simulink model "ALU"  (R2021a)
settings: Solver=VariableStepAuto  StartTime=0.0  StopTime=10.0  RelTol=1e-3
settings Model: Creator=kbhar  LastModifiedBy=kbhar

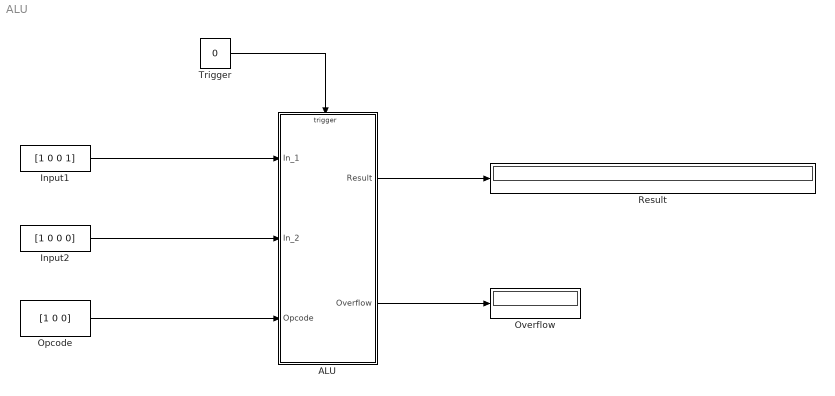
== system ALU ==
  ALU : Subsystem
  Input1 : Constant  Value=[1 0 0 1]
  Input2 : Constant  Value=[1 0 0 0]
  Opcode : Constant  Value=[1 0 0]
  Overflow : Display
  Result : Display
  Trigger : Constant  Value=0
  wires:
  Input2/1 -> ALU/2(In_2)
  Input1/1 -> ALU/1(In_1)
  Opcode/1 -> ALU/3(Opcode)
  ALU/1(Result) -> Result/1
  ALU/2(Overflow) -> Overflow/1
  Trigger/1 -> ALU/Trigger

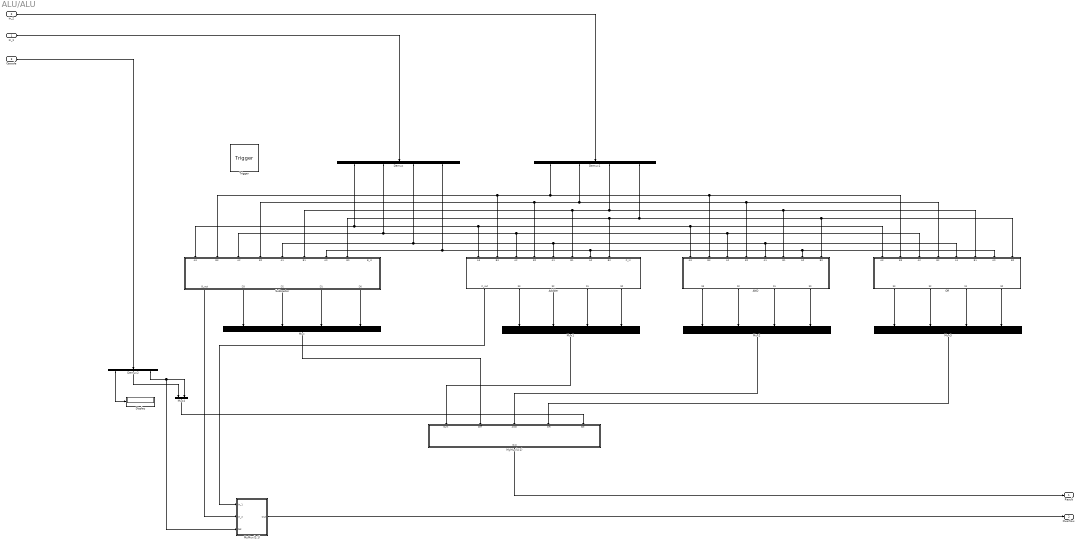
== system ALU/ALU ==
  In_1 : Inport
  In_2 : Inport  Port=2
  Opcode : Inport  Port=3
  Trigger : TriggerPort  VariantControl=(inherit)  PortDimensions=1
  AND : Subsystem
  Addder : Subsystem
  Demux : Demux
  Demux1 : Demux
  Demux2 : Demux  Outputs=3
  Display : Display
  Mux{,1..3} (4 alike) : Mux
  Mux4 : Mux  Inputs=2
  MyMux(2:1) : Subsystem
  MyMux(4:1) : Subsystem
  OR : Subsystem
  Subtractor : Subsystem
  Result : Outport
  Overflow : Outport  Port=2
  wires:
  AND/2(S2) -> Mux2/2
  Demux1/3 -> OR/6(B1), AND/6(B1), Subtractor/6(B1), Addder/6(B1)
  OR/1(S3) -> Mux3/1
  Subtractor/5(D0) -> Mux/4
  OR/3(S1) -> Mux3/3
  Demux1/2 -> OR/4(B2), AND/4(B2), Subtractor/4(B2), Addder/4(B2)
  Mux/1 -> MyMux(4:1)/2(Diff)
  Demux/4 -> Subtractor/7(A0), OR/7(A0), AND/7(A0), Addder/7(A0)
  Addder/3(S2) -> Mux1/2
  Subtractor/2(D3) -> Mux/1
  Demux1/4 -> Subtractor/8(B0), Addder/8(B0), OR/8(B0), AND/8(B0)
  Demux/2 -> Subtractor/3(A2), OR/3(A2), AND/3(A2), Addder/3(A2)
  Demux/1 -> Subtractor/1(A3), OR/1(A3), AND/1(A3), Addder/1(A3)
  MyMux(2:1)/1(Out) -> Overflow/1
  Subtractor/1(B_out) -> MyMux(2:1)/2(In_2)
  Demux1/1 -> OR/2(B3), AND/2(B3), Subtractor/2(B3), Addder/2(B3)
  Demux/3 -> Subtractor/5(A1), AND/5(A1), OR/5(A1), Addder/5(A1)
  MyMux(4:1)/1(Out) -> Result/1
  Subtractor/3(D2) -> Mux/2
  Mux3/1 -> MyMux(4:1)/4(OR)
  Subtractor/4(D1) -> Mux/3
  Mux1/1 -> MyMux(4:1)/1(Sum)
  ? -> Addder/9(C_in)
  AND/1(S3) -> Mux2/1
  Mux2/1 -> MyMux(4:1)/3(AND)
  In_2/1 -> Demux1/1
  OR/2(S2) -> Mux3/2
  Mux4/1 -> MyMux(4:1)/5(Sel)
  AND/4(S0) -> Mux2/4
  Demux2/1 -> Display/1
  Demux2/3 -> MyMux(2:1)/3(Sel), Mux4/2
  Demux2/2 -> Mux4/1
  Addder/1(C_out) -> MyMux(2:1)/1(In_1)
  Addder/4(S1) -> Mux1/3
  AND/3(S1) -> Mux2/3
  Addder/5(S0) -> Mux1/4
  OR/4(S0) -> Mux3/4
  ? -> Subtractor/9(B_in)
  Addder/2(S3) -> Mux1/1
  Opcode/1 -> Demux2/1
  In_1/1 -> Demux/1

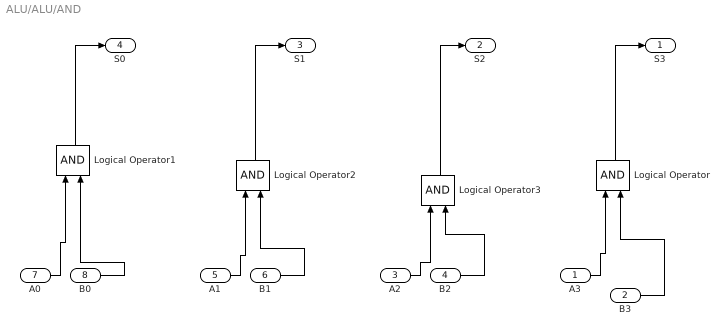
== system ALU/ALU/AND ==
  A3 : Inport
  B3 : Inport  Port=2
  A2 : Inport  Port=3
  B2 : Inport  Port=4
  A1 : Inport  Port=5
  B1 : Inport  Port=6
  A0 : Inport  Port=7
  B0 : Inport  Port=8
  Logical Operator{,1..3} (4 alike) : Logic  AllPortsSameDT=off  OutDataTypeStr=boolean
  S3 : Outport
  S2 : Outport  Port=2
  S1 : Outport  Port=3
  S0 : Outport  Port=4
  wires:
  Logical Operator2/1 -> S1/1
  B1/1 -> Logical Operator2/2
  A1/1 -> Logical Operator2/1
  A2/1 -> Logical Operator3/1
  B0/1 -> Logical Operator1/2
  B3/1 -> Logical Operator/2
  B2/1 -> Logical Operator3/2
  A0/1 -> Logical Operator1/1
  A3/1 -> Logical Operator/1
  Logical Operator3/1 -> S2/1
  Logical Operator1/1 -> S0/1
  Logical Operator/1 -> S3/1

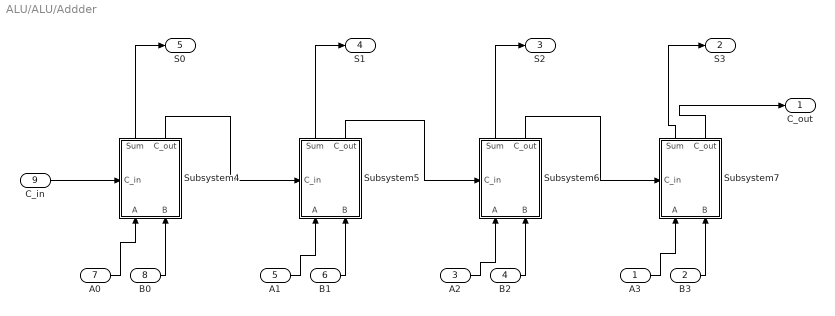
== system ALU/ALU/Addder ==
  A3 : Inport
  B3 : Inport  Port=2
  A2 : Inport  Port=3
  B2 : Inport  Port=4
  A1 : Inport  Port=5
  B1 : Inport  Port=6
  A0 : Inport  Port=7
  B0 : Inport  Port=8
  C_in : Inport  Port=9
  Subsystem4 : Subsystem
      settings: PortSchema="{\"entries\":[{\"content\":{\"sides\":[{\"content\":{\"connectorIds\":[\"In1\",\"In2\"]},\"type\":\"ConnectorPlacement.EquallySpacedRectSide\",\"uuid\":\"38d1d783-1e84-469f-b88f-34400794f458\"},{\"content\":{\"connectorIds\":[\"Out1\",\"Out2\"],\"side\":\"RIGHT\"},\"type\":\"ConnectorPlacement.EquallySpacedRectSide\",\"uuid\":\"9549b396-3b16-432f-9c12-dae7a5b8dc11\"},{\"content\":{\"connectorIds\":[\"In3\"],\"side\":\"TOP\"},\"type\":\"ConnectorPlacement.EquallySpacedRectSide\",\"uuid\":\"526a5790-86b3-4626-b4aa-b9520108ec40\"}]},\"type\":\"ConnectorPlacement.EquallySpacedConnector\",\"uuid\":\"b57ea0ad-738f-4734-9daa-a65058de1f48\"}],\"packageUris\":[\"http://schema.mathworks.com/mf0/Connector/R2020b\"],\"version\":\"1.0\"}"
  Subsystem5 : Subsystem
      settings: PortSchema="{\"entries\":[{\"content\":{\"sides\":[{\"content\":{\"connectorIds\":[\"In1\",\"In2\"]},\"type\":\"ConnectorPlacement.EquallySpacedRectSide\",\"uuid\":\"38d1d783-1e84-469f-b88f-34400794f458\"},{\"content\":{\"connectorIds\":[\"Out1\",\"Out2\"],\"side\":\"RIGHT\"},\"type\":\"ConnectorPlacement.EquallySpacedRectSide\",\"uuid\":\"9549b396-3b16-432f-9c12-dae7a5b8dc11\"},{\"content\":{\"connectorIds\":[\"In3\"],\"side\":\"TOP\"},\"type\":\"ConnectorPlacement.EquallySpacedRectSide\",\"uuid\":\"526a5790-86b3-4626-b4aa-b9520108ec40\"}]},\"type\":\"ConnectorPlacement.EquallySpacedConnector\",\"uuid\":\"b57ea0ad-738f-4734-9daa-a65058de1f48\"}],\"packageUris\":[\"http://schema.mathworks.com/mf0/Connector/R2020b\"],\"version\":\"1.0\"}"
  Subsystem6 : Subsystem
      settings: PortSchema="{\"entries\":[{\"content\":{\"sides\":[{\"content\":{\"connectorIds\":[\"In1\",\"In2\"]},\"type\":\"ConnectorPlacement.EquallySpacedRectSide\",\"uuid\":\"38d1d783-1e84-469f-b88f-34400794f458\"},{\"content\":{\"connectorIds\":[\"Out1\",\"Out2\"],\"side\":\"RIGHT\"},\"type\":\"ConnectorPlacement.EquallySpacedRectSide\",\"uuid\":\"9549b396-3b16-432f-9c12-dae7a5b8dc11\"},{\"content\":{\"connectorIds\":[\"In3\"],\"side\":\"TOP\"},\"type\":\"ConnectorPlacement.EquallySpacedRectSide\",\"uuid\":\"526a5790-86b3-4626-b4aa-b9520108ec40\"}]},\"type\":\"ConnectorPlacement.EquallySpacedConnector\",\"uuid\":\"b57ea0ad-738f-4734-9daa-a65058de1f48\"}],\"packageUris\":[\"http://schema.mathworks.com/mf0/Connector/R2020b\"],\"version\":\"1.0\"}"
  Subsystem7 : Subsystem
      settings: PortSchema="{\"entries\":[{\"content\":{\"sides\":[{\"content\":{\"connectorIds\":[\"In1\",\"In2\"]},\"type\":\"ConnectorPlacement.EquallySpacedRectSide\",\"uuid\":\"38d1d783-1e84-469f-b88f-34400794f458\"},{\"content\":{\"connectorIds\":[\"Out1\",\"Out2\"],\"side\":\"RIGHT\"},\"type\":\"ConnectorPlacement.EquallySpacedRectSide\",\"uuid\":\"9549b396-3b16-432f-9c12-dae7a5b8dc11\"},{\"content\":{\"connectorIds\":[\"In3\"],\"side\":\"TOP\"},\"type\":\"ConnectorPlacement.EquallySpacedRectSide\",\"uuid\":\"526a5790-86b3-4626-b4aa-b9520108ec40\"}]},\"type\":\"ConnectorPlacement.EquallySpacedConnector\",\"uuid\":\"b57ea0ad-738f-4734-9daa-a65058de1f48\"}],\"packageUris\":[\"http://schema.mathworks.com/mf0/Connector/R2020b\"],\"version\":\"1.0\"}"
  C_out : Outport
  S3 : Outport  Port=2
  S2 : Outport  Port=3
  S1 : Outport  Port=4
  S0 : Outport  Port=5
  wires:
  Subsystem5/2(C_out) -> Subsystem6/3(C_in)
  Subsystem5/1(Sum) -> S1/1
  Subsystem7/2(C_out) -> C_out/1
  B1/1 -> Subsystem5/2(B)
  Subsystem6/2(C_out) -> Subsystem7/3(C_in)
  A1/1 -> Subsystem5/1(A)
  A2/1 -> Subsystem6/1(A)
  Subsystem4/2(C_out) -> Subsystem5/3(C_in)
  B0/1 -> Subsystem4/2(B)
  B3/1 -> Subsystem7/2(B)
  B2/1 -> Subsystem6/2(B)
  A0/1 -> Subsystem4/1(A)
  A3/1 -> Subsystem7/1(A)
  Subsystem6/1(Sum) -> S2/1
  C_in/1 -> Subsystem4/3(C_in)
  Subsystem4/1(Sum) -> S0/1
  Subsystem7/1(Sum) -> S3/1

== system ALU/ALU/MyMux(2:1) ==
  In_1 : Inport
  In_2 : Inport  Port=2
  Sel : Inport  Port=3
  Logical Operator : Logic  AllPortsSameDT=off  OutDataTypeStr=boolean
  Logical Operator1 : Logic  Operator=NOT  AllPortsSameDT=off  OutDataTypeStr=boolean
  Logical Operator2 : Logic  AllPortsSameDT=off  OutDataTypeStr=boolean
  Logical Operator3 : Logic  Operator=OR  AllPortsSameDT=off  OutDataTypeStr=boolean
  Out : Outport
  wires:
  Logical Operator1/1 -> Logical Operator/2
  In_1/1 -> Logical Operator/1
  Logical Operator2/1 -> Logical Operator3/2
  Sel/1 -> Logical Operator1/1, Logical Operator2/2
  Logical Operator3/1 -> Out/1
  In_2/1 -> Logical Operator2/1
  Logical Operator/1 -> Logical Operator3/1

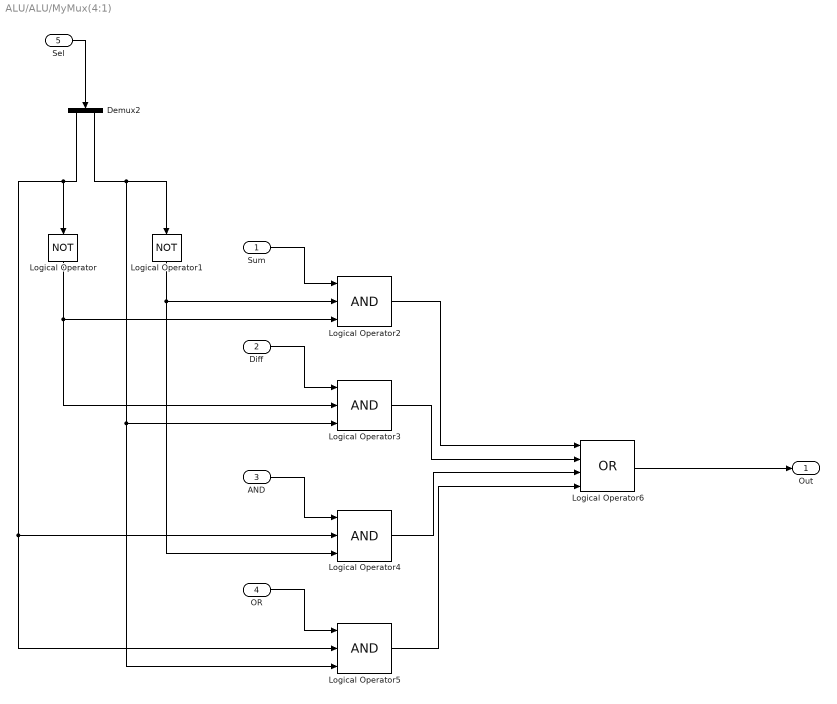
== system ALU/ALU/MyMux(4:1) ==
  Sum : Inport
  Diff : Inport  Port=2
  AND : Inport  Port=3
  OR : Inport  Port=4
  Sel : Inport  Port=5
  Demux2 : Demux  Outputs=2
  Logical Operator : Logic  Operator=NOT  AllPortsSameDT=off  OutDataTypeStr=boolean
  Logical Operator1 : Logic  Operator=NOT  AllPortsSameDT=off  OutDataTypeStr=boolean
  Logical Operator{2..5} (4 alike) : Logic  Inputs=3  AllPortsSameDT=off  OutDataTypeStr=boolean
  Logical Operator6 : Logic  Operator=OR  Inputs=4  AllPortsSameDT=off  OutDataTypeStr=boolean
  Out : Outport
  wires:
  Demux2/1 -> Logical Operator4/2, Logical Operator5/2, Logical Operator/1
  Demux2/2 -> Logical Operator5/3, Logical Operator3/3, Logical Operator1/1
  Logical Operator1/1 -> Logical Operator2/2, Logical Operator4/3
  Logical Operator2/1 -> Logical Operator6/1
  Logical Operator3/1 -> Logical Operator6/2
  Logical Operator/1 -> Logical Operator2/3, Logical Operator3/2
  Logical Operator4/1 -> Logical Operator6/3
  Logical Operator5/1 -> Logical Operator6/4
  Diff/1 -> Logical Operator3/1
  AND/1 -> Logical Operator4/1
  OR/1 -> Logical Operator5/1
  Sum/1 -> Logical Operator2/1
  Logical Operator6/1 -> Out/1
  Sel/1 -> Demux2/1

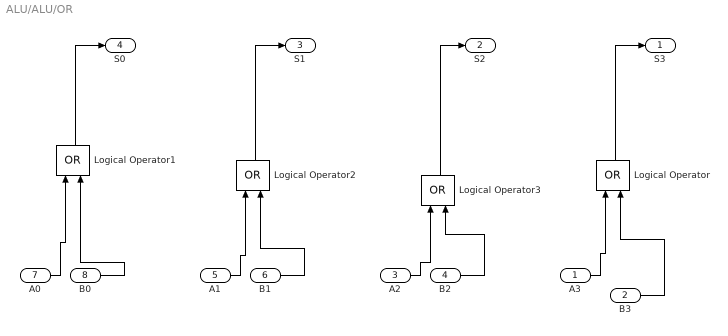
== system ALU/ALU/OR ==
  A3 : Inport
  B3 : Inport  Port=2
  A2 : Inport  Port=3
  B2 : Inport  Port=4
  A1 : Inport  Port=5
  B1 : Inport  Port=6
  A0 : Inport  Port=7
  B0 : Inport  Port=8
  Logical Operator{,1..3} (4 alike) : Logic  Operator=OR  AllPortsSameDT=off  OutDataTypeStr=boolean
  S3 : Outport
  S2 : Outport  Port=2
  S1 : Outport  Port=3
  S0 : Outport  Port=4
  wires:
  Logical Operator2/1 -> S1/1
  B1/1 -> Logical Operator2/2
  A1/1 -> Logical Operator2/1
  A2/1 -> Logical Operator3/1
  B0/1 -> Logical Operator1/2
  B3/1 -> Logical Operator/2
  B2/1 -> Logical Operator3/2
  A0/1 -> Logical Operator1/1
  A3/1 -> Logical Operator/1
  Logical Operator3/1 -> S2/1
  Logical Operator1/1 -> S0/1
  Logical Operator/1 -> S3/1

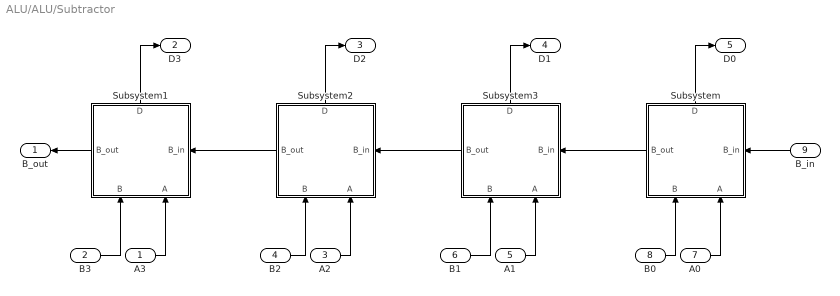
== system ALU/ALU/Subtractor ==
  A3 : Inport
  B3 : Inport  Port=2
  A2 : Inport  Port=3
  B2 : Inport  Port=4
  A1 : Inport  Port=5
  B1 : Inport  Port=6
  A0 : Inport  Port=7
  B0 : Inport  Port=8
  B_in : Inport  Port=9
  Subsystem : Subsystem
      settings: PortSchema="{\"entries\":[{\"content\":{\"sides\":[{\"content\":{\"connectorIds\":[\"In1\",\"In2\"]},\"type\":\"ConnectorPlacement.EquallySpacedRectSide\",\"uuid\":\"38d1d783-1e84-469f-b88f-34400794f458\"},{\"content\":{\"connectorIds\":[\"Out1\"],\"side\":\"RIGHT\"},\"type\":\"ConnectorPlacement.EquallySpacedRectSide\",\"uuid\":\"9549b396-3b16-432f-9c12-dae7a5b8dc11\"},{\"content\":{\"connectorIds\":[\"Out2\"],\"side\":\"TOP\"},\"type\":\"ConnectorPlacement.EquallySpacedRectSide\",\"uuid\":\"526a5790-86b3-4626-b4aa-b9520108ec40\"},{\"content\":{\"connectorIds\":[\"In3\"],\"side\":\"BOTTOM\"},\"type\":\"ConnectorPlacement.EquallySpacedRectSide\",\"uuid\":\"7b9a1b6a-14be-425f-b6da-6563ee756159\"}]},\"type\":\"ConnectorPlacement.EquallySpacedConnector\",\"uuid\":\"b57ea0ad-738f-4734-9daa-a65058de1f48\"}],\"packageUris\":[\"http://schema.mathworks.com/mf0/Connector/R2020b\"],\"version\":\"1.0\"}"
  Subsystem1 : Subsystem
      settings: PortSchema="{\"entries\":[{\"content\":{\"sides\":[{\"content\":{\"connectorIds\":[\"In1\",\"In2\"]},\"type\":\"ConnectorPlacement.EquallySpacedRectSide\",\"uuid\":\"38d1d783-1e84-469f-b88f-34400794f458\"},{\"content\":{\"connectorIds\":[\"Out1\"],\"side\":\"RIGHT\"},\"type\":\"ConnectorPlacement.EquallySpacedRectSide\",\"uuid\":\"9549b396-3b16-432f-9c12-dae7a5b8dc11\"},{\"content\":{\"connectorIds\":[\"Out2\"],\"side\":\"TOP\"},\"type\":\"ConnectorPlacement.EquallySpacedRectSide\",\"uuid\":\"526a5790-86b3-4626-b4aa-b9520108ec40\"},{\"content\":{\"connectorIds\":[\"In3\"],\"side\":\"BOTTOM\"},\"type\":\"ConnectorPlacement.EquallySpacedRectSide\",\"uuid\":\"7b9a1b6a-14be-425f-b6da-6563ee756159\"}]},\"type\":\"ConnectorPlacement.EquallySpacedConnector\",\"uuid\":\"b57ea0ad-738f-4734-9daa-a65058de1f48\"}],\"packageUris\":[\"http://schema.mathworks.com/mf0/Connector/R2020b\"],\"version\":\"1.0\"}"
  Subsystem2 : Subsystem
      settings: PortSchema="{\"entries\":[{\"content\":{\"sides\":[{\"content\":{\"connectorIds\":[\"In1\",\"In2\"]},\"type\":\"ConnectorPlacement.EquallySpacedRectSide\",\"uuid\":\"38d1d783-1e84-469f-b88f-34400794f458\"},{\"content\":{\"connectorIds\":[\"Out1\"],\"side\":\"RIGHT\"},\"type\":\"ConnectorPlacement.EquallySpacedRectSide\",\"uuid\":\"9549b396-3b16-432f-9c12-dae7a5b8dc11\"},{\"content\":{\"connectorIds\":[\"Out2\"],\"side\":\"TOP\"},\"type\":\"ConnectorPlacement.EquallySpacedRectSide\",\"uuid\":\"526a5790-86b3-4626-b4aa-b9520108ec40\"},{\"content\":{\"connectorIds\":[\"In3\"],\"side\":\"BOTTOM\"},\"type\":\"ConnectorPlacement.EquallySpacedRectSide\",\"uuid\":\"7b9a1b6a-14be-425f-b6da-6563ee756159\"}]},\"type\":\"ConnectorPlacement.EquallySpacedConnector\",\"uuid\":\"b57ea0ad-738f-4734-9daa-a65058de1f48\"}],\"packageUris\":[\"http://schema.mathworks.com/mf0/Connector/R2020b\"],\"version\":\"1.0\"}"
  Subsystem3 : Subsystem
      settings: PortSchema="{\"entries\":[{\"content\":{\"sides\":[{\"content\":{\"connectorIds\":[\"In1\",\"In2\"]},\"type\":\"ConnectorPlacement.EquallySpacedRectSide\",\"uuid\":\"38d1d783-1e84-469f-b88f-34400794f458\"},{\"content\":{\"connectorIds\":[\"Out1\"],\"side\":\"RIGHT\"},\"type\":\"ConnectorPlacement.EquallySpacedRectSide\",\"uuid\":\"9549b396-3b16-432f-9c12-dae7a5b8dc11\"},{\"content\":{\"connectorIds\":[\"Out2\"],\"side\":\"TOP\"},\"type\":\"ConnectorPlacement.EquallySpacedRectSide\",\"uuid\":\"526a5790-86b3-4626-b4aa-b9520108ec40\"},{\"content\":{\"connectorIds\":[\"In3\"],\"side\":\"BOTTOM\"},\"type\":\"ConnectorPlacement.EquallySpacedRectSide\",\"uuid\":\"7b9a1b6a-14be-425f-b6da-6563ee756159\"}]},\"type\":\"ConnectorPlacement.EquallySpacedConnector\",\"uuid\":\"b57ea0ad-738f-4734-9daa-a65058de1f48\"}],\"packageUris\":[\"http://schema.mathworks.com/mf0/Connector/R2020b\"],\"version\":\"1.0\"}"
  B_out : Outport
  D3 : Outport  Port=2
  D2 : Outport  Port=3
  D1 : Outport  Port=4
  D0 : Outport  Port=5
  wires:
  B_in/1 -> Subsystem/3(B_in)
  Subsystem3/2(B_out) -> Subsystem2/3(B_in)
  Subsystem2/2(B_out) -> Subsystem1/3(B_in)
  Subsystem/2(B_out) -> Subsystem3/3(B_in)
  Subsystem1/2(B_out) -> B_out/1
  A0/1 -> Subsystem/2(A)
  B0/1 -> Subsystem/1(B)
  B3/1 -> Subsystem1/1(B)
  A3/1 -> Subsystem1/2(A)
  A1/1 -> Subsystem3/2(A)
  B1/1 -> Subsystem3/1(B)
  B2/1 -> Subsystem2/1(B)
  A2/1 -> Subsystem2/2(A)
  Subsystem1/1(D) -> D3/1
  Subsystem/1(D) -> D0/1
  Subsystem3/1(D) -> D1/1
  Subsystem2/1(D) -> D2/1

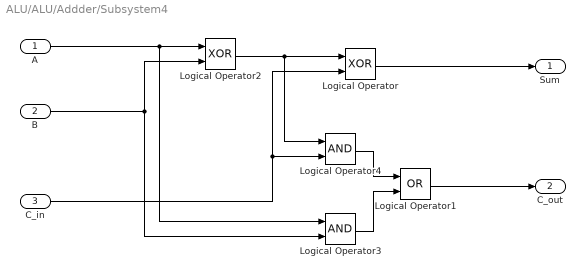
== system ALU/ALU/Addder/Subsystem4 ==
  A : Inport
  B : Inport  Port=2
  C_in : Inport  Port=3
  Logical Operator : Logic  Operator=XOR  AllPortsSameDT=off  OutDataTypeStr=boolean
  Logical Operator1 : Logic  Operator=OR  AllPortsSameDT=off  OutDataTypeStr=boolean
  Logical Operator2 : Logic  Operator=XOR  AllPortsSameDT=off  OutDataTypeStr=boolean
  Logical Operator3 : Logic  AllPortsSameDT=off  OutDataTypeStr=boolean
  Logical Operator4 : Logic  AllPortsSameDT=off  OutDataTypeStr=boolean
  Sum : Outport
  C_out : Outport  Port=2
  wires:
  B/1 -> Logical Operator3/2, Logical Operator2/2
  A/1 -> Logical Operator3/1, Logical Operator2/1
  Logical Operator4/1 -> Logical Operator1/1
  Logical Operator/1 -> Sum/1
  Logical Operator2/1 -> Logical Operator4/1, Logical Operator/1
  C_in/1 -> Logical Operator4/2, Logical Operator/2
  Logical Operator3/1 -> Logical Operator1/2
  Logical Operator1/1 -> C_out/1

== system ALU/ALU/Addder/Subsystem5 ==
  A : Inport
  B : Inport  Port=2
  C_in : Inport  Port=3
  Logical Operator : Logic  Operator=XOR  AllPortsSameDT=off  OutDataTypeStr=boolean
  Logical Operator1 : Logic  Operator=OR  AllPortsSameDT=off  OutDataTypeStr=boolean
  Logical Operator2 : Logic  Operator=XOR  AllPortsSameDT=off  OutDataTypeStr=boolean
  Logical Operator3 : Logic  AllPortsSameDT=off  OutDataTypeStr=boolean
  Logical Operator4 : Logic  AllPortsSameDT=off  OutDataTypeStr=boolean
  Sum : Outport
  C_out : Outport  Port=2
  wires:
  B/1 -> Logical Operator3/2, Logical Operator2/2
  A/1 -> Logical Operator3/1, Logical Operator2/1
  Logical Operator4/1 -> Logical Operator1/1
  Logical Operator/1 -> Sum/1
  Logical Operator2/1 -> Logical Operator4/1, Logical Operator/1
  C_in/1 -> Logical Operator4/2, Logical Operator/2
  Logical Operator3/1 -> Logical Operator1/2
  Logical Operator1/1 -> C_out/1

== system ALU/ALU/Addder/Subsystem6 ==
  A : Inport
  B : Inport  Port=2
  C_in : Inport  Port=3
  Logical Operator : Logic  Operator=XOR  AllPortsSameDT=off  OutDataTypeStr=boolean
  Logical Operator1 : Logic  Operator=OR  AllPortsSameDT=off  OutDataTypeStr=boolean
  Logical Operator2 : Logic  Operator=XOR  AllPortsSameDT=off  OutDataTypeStr=boolean
  Logical Operator3 : Logic  AllPortsSameDT=off  OutDataTypeStr=boolean
  Logical Operator4 : Logic  AllPortsSameDT=off  OutDataTypeStr=boolean
  Sum : Outport
  C_out : Outport  Port=2
  wires:
  B/1 -> Logical Operator3/2, Logical Operator2/2
  A/1 -> Logical Operator3/1, Logical Operator2/1
  Logical Operator4/1 -> Logical Operator1/1
  Logical Operator/1 -> Sum/1
  Logical Operator2/1 -> Logical Operator4/1, Logical Operator/1
  C_in/1 -> Logical Operator4/2, Logical Operator/2
  Logical Operator3/1 -> Logical Operator1/2
  Logical Operator1/1 -> C_out/1

== system ALU/ALU/Addder/Subsystem7 ==
  A : Inport
  B : Inport  Port=2
  C_in : Inport  Port=3
  Logical Operator : Logic  Operator=XOR  AllPortsSameDT=off  OutDataTypeStr=boolean
  Logical Operator1 : Logic  Operator=OR  AllPortsSameDT=off  OutDataTypeStr=boolean
  Logical Operator2 : Logic  Operator=XOR  AllPortsSameDT=off  OutDataTypeStr=boolean
  Logical Operator3 : Logic  AllPortsSameDT=off  OutDataTypeStr=boolean
  Logical Operator4 : Logic  AllPortsSameDT=off  OutDataTypeStr=boolean
  Sum : Outport
  C_out : Outport  Port=2
  wires:
  B/1 -> Logical Operator3/2, Logical Operator2/2
  A/1 -> Logical Operator3/1, Logical Operator2/1
  Logical Operator4/1 -> Logical Operator1/1
  Logical Operator/1 -> Sum/1
  Logical Operator2/1 -> Logical Operator4/1, Logical Operator/1
  C_in/1 -> Logical Operator4/2, Logical Operator/2
  Logical Operator3/1 -> Logical Operator1/2
  Logical Operator1/1 -> C_out/1

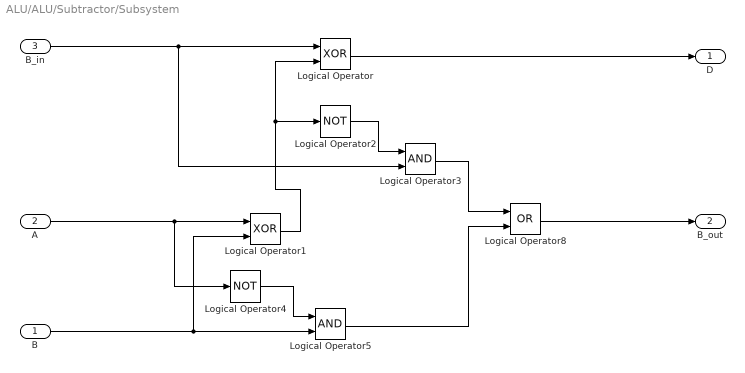
== system ALU/ALU/Subtractor/Subsystem ==
  B : Inport
  A : Inport  Port=2
  B_in : Inport  Port=3
  Logical Operator : Logic  Operator=XOR  AllPortsSameDT=off  OutDataTypeStr=boolean
  Logical Operator1 : Logic  Operator=XOR  AllPortsSameDT=off  OutDataTypeStr=boolean
  Logical Operator2 : Logic  Operator=NOT  AllPortsSameDT=off  OutDataTypeStr=boolean
  Logical Operator3 : Logic  AllPortsSameDT=off  OutDataTypeStr=boolean
  Logical Operator4 : Logic  Operator=NOT  AllPortsSameDT=off  OutDataTypeStr=boolean
  Logical Operator5 : Logic  AllPortsSameDT=off  OutDataTypeStr=boolean
  Logical Operator8 : Logic  Operator=OR  AllPortsSameDT=off  OutDataTypeStr=boolean
  D : Outport
  B_out : Outport  Port=2
  wires:
  Logical Operator2/1 -> Logical Operator3/1
  B_in/1 -> Logical Operator/1, Logical Operator3/2
  B/1 -> Logical Operator1/2, Logical Operator5/2
  Logical Operator1/1 -> Logical Operator2/1, Logical Operator/2
  A/1 -> Logical Operator1/1, Logical Operator4/1
  Logical Operator3/1 -> Logical Operator8/1
  Logical Operator5/1 -> Logical Operator8/2
  Logical Operator4/1 -> Logical Operator5/1
  Logical Operator/1 -> D/1
  Logical Operator8/1 -> B_out/1

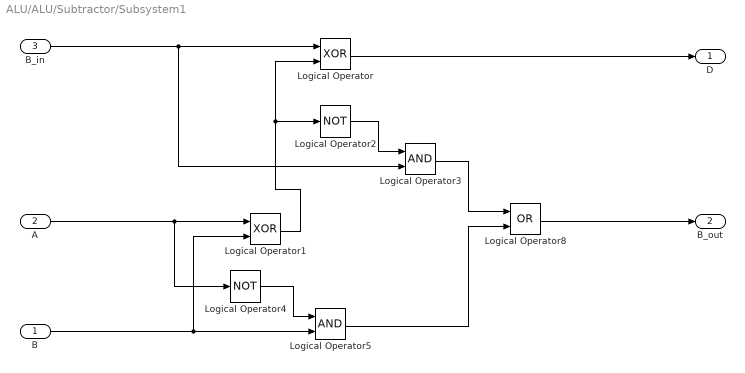
== system ALU/ALU/Subtractor/Subsystem1 ==
  B : Inport
  A : Inport  Port=2
  B_in : Inport  Port=3
  Logical Operator : Logic  Operator=XOR  AllPortsSameDT=off  OutDataTypeStr=boolean
  Logical Operator1 : Logic  Operator=XOR  AllPortsSameDT=off  OutDataTypeStr=boolean
  Logical Operator2 : Logic  Operator=NOT  AllPortsSameDT=off  OutDataTypeStr=boolean
  Logical Operator3 : Logic  AllPortsSameDT=off  OutDataTypeStr=boolean
  Logical Operator4 : Logic  Operator=NOT  AllPortsSameDT=off  OutDataTypeStr=boolean
  Logical Operator5 : Logic  AllPortsSameDT=off  OutDataTypeStr=boolean
  Logical Operator8 : Logic  Operator=OR  AllPortsSameDT=off  OutDataTypeStr=boolean
  D : Outport
  B_out : Outport  Port=2
  wires:
  Logical Operator2/1 -> Logical Operator3/1
  B_in/1 -> Logical Operator/1, Logical Operator3/2
  B/1 -> Logical Operator1/2, Logical Operator5/2
  Logical Operator1/1 -> Logical Operator2/1, Logical Operator/2
  A/1 -> Logical Operator1/1, Logical Operator4/1
  Logical Operator3/1 -> Logical Operator8/1
  Logical Operator5/1 -> Logical Operator8/2
  Logical Operator4/1 -> Logical Operator5/1
  Logical Operator/1 -> D/1
  Logical Operator8/1 -> B_out/1

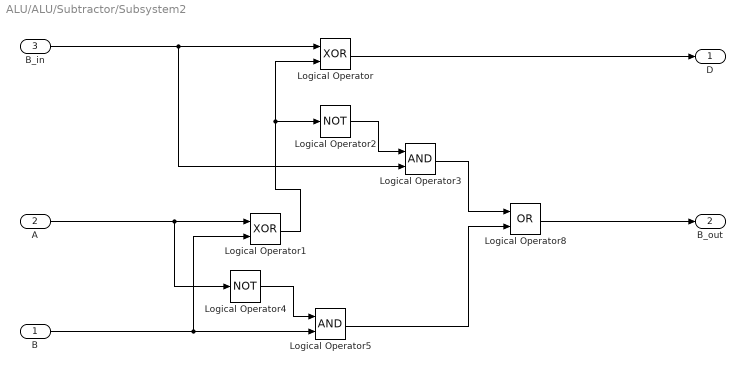
== system ALU/ALU/Subtractor/Subsystem2 ==
  B : Inport
  A : Inport  Port=2
  B_in : Inport  Port=3
  Logical Operator : Logic  Operator=XOR  AllPortsSameDT=off  OutDataTypeStr=boolean
  Logical Operator1 : Logic  Operator=XOR  AllPortsSameDT=off  OutDataTypeStr=boolean
  Logical Operator2 : Logic  Operator=NOT  AllPortsSameDT=off  OutDataTypeStr=boolean
  Logical Operator3 : Logic  AllPortsSameDT=off  OutDataTypeStr=boolean
  Logical Operator4 : Logic  Operator=NOT  AllPortsSameDT=off  OutDataTypeStr=boolean
  Logical Operator5 : Logic  AllPortsSameDT=off  OutDataTypeStr=boolean
  Logical Operator8 : Logic  Operator=OR  AllPortsSameDT=off  OutDataTypeStr=boolean
  D : Outport
  B_out : Outport  Port=2
  wires:
  Logical Operator2/1 -> Logical Operator3/1
  B_in/1 -> Logical Operator/1, Logical Operator3/2
  B/1 -> Logical Operator1/2, Logical Operator5/2
  Logical Operator1/1 -> Logical Operator2/1, Logical Operator/2
  A/1 -> Logical Operator1/1, Logical Operator4/1
  Logical Operator3/1 -> Logical Operator8/1
  Logical Operator5/1 -> Logical Operator8/2
  Logical Operator4/1 -> Logical Operator5/1
  Logical Operator/1 -> D/1
  Logical Operator8/1 -> B_out/1

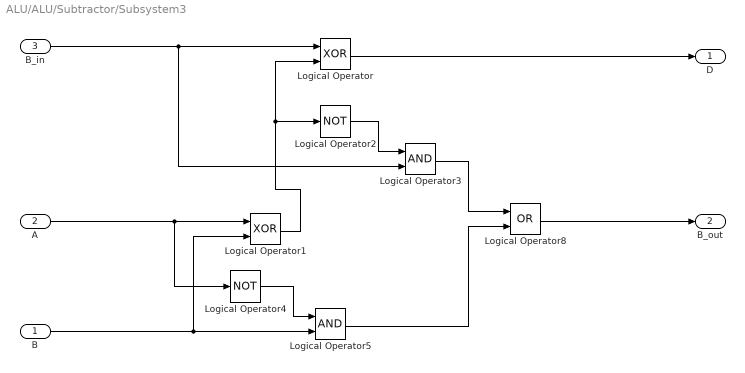
== system ALU/ALU/Subtractor/Subsystem3 ==
  B : Inport
  A : Inport  Port=2
  B_in : Inport  Port=3
  Logical Operator : Logic  Operator=XOR  AllPortsSameDT=off  OutDataTypeStr=boolean
  Logical Operator1 : Logic  Operator=XOR  AllPortsSameDT=off  OutDataTypeStr=boolean
  Logical Operator2 : Logic  Operator=NOT  AllPortsSameDT=off  OutDataTypeStr=boolean
  Logical Operator3 : Logic  AllPortsSameDT=off  OutDataTypeStr=boolean
  Logical Operator4 : Logic  Operator=NOT  AllPortsSameDT=off  OutDataTypeStr=boolean
  Logical Operator5 : Logic  AllPortsSameDT=off  OutDataTypeStr=boolean
  Logical Operator8 : Logic  Operator=OR  AllPortsSameDT=off  OutDataTypeStr=boolean
  D : Outport
  B_out : Outport  Port=2
  wires:
  Logical Operator2/1 -> Logical Operator3/1
  B_in/1 -> Logical Operator/1, Logical Operator3/2
  B/1 -> Logical Operator1/2, Logical Operator5/2
  Logical Operator1/1 -> Logical Operator2/1, Logical Operator/2
  A/1 -> Logical Operator1/1, Logical Operator4/1
  Logical Operator3/1 -> Logical Operator8/1
  Logical Operator5/1 -> Logical Operator8/2
  Logical Operator4/1 -> Logical Operator5/1
  Logical Operator/1 -> D/1
  Logical Operator8/1 -> B_out/1
